simulink model "ExplicacionMatlabFunction"  (R2017b)
settings: Solver=VariableStepAuto  StartTime=0.0  StopTime=10  RelTol=1e-3
settings Model: Creator=Cx001la  LastModifiedBy=Cx001la

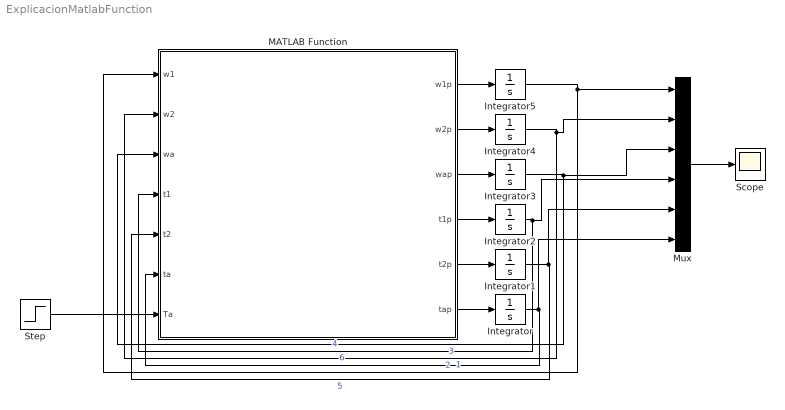
== system ExplicacionMatlabFunction ==
  Integrator{,1..5} (6 alike) : Integrator
  MATLAB Function : MATLAB Function  TreatAsAtomicUnit=on
  Mux : Mux  Inputs=6
  Scope : Scope
  Step : Step  Time=0  SampleTime=0
  wires:
  MATLAB Function/1(w1p) -> Integrator5/1
  MATLAB Function/2(w2p) -> Integrator4/1
  MATLAB Function/3(wap) -> Integrator3/1
  MATLAB Function/4(t1p) -> Integrator2/1
  MATLAB Function/5(t2p) -> Integrator1/1
  MATLAB Function/6(tap) -> Integrator/1
  Integrator/1 -> Mux/6, MATLAB Function/6(ta)  "6"
  Integrator1/1 -> Mux/5, MATLAB Function/5(t2)  "5"
  Integrator2/1 -> Mux/4, MATLAB Function/4(t1)  "4"
  Integrator3/1 -> Mux/3, MATLAB Function/3(wa)  "3"
  Integrator4/1 -> Mux/2, MATLAB Function/2(w2)  "2"
  Integrator5/1 -> Mux/1, MATLAB Function/1(w1)  "1"
  Step/1 -> MATLAB Function/7(Ta)
  Mux/1 -> Scope/1

== matlab function ExplicacionMatlabFunction/MATLAB Function ==
  data: w1 input; w1p output; w2 input; wa input; t1 input; t2 input; ta input; Ta input; w2p output; wap output; t1p output; t2p output; tap output
function [w1p, w2p, wap, t1p, t2p, tap] = ftp2(w1,w2,wa,t1,t2,ta,Ta)

j1=0.625; j2=1.08; ja=0.135; jb=0.04; r1=0.5; r2=0.6; ra=0.3; rb=0.2; k1=100; k2=250; b1=10; b2=15; %Constantes

TL=5*w2*abs(w2);
w1p=(Ta-b1*w1-k1*(t1-ta) )/j1;
w2p=(k2*(ta*ra/rb-t2) - b2*t2-TL )/j2;
wap=(rb*rb*k1/(ja*rb*rb+jb*ra*ra)   )*(t1-ta);
t1p=w1;
t2p=w2;
tap=wa;
